simulink model "test_modello"  (R2023a)
settings: Solver=FixedStepAuto  StartTime=0.0  StopTime=50  FixedStep=0.01  RelTol=1e-3
settings Model: PacingRate=0.500000  Creator=kiraa  LastModifiedBy=david
settings OptimizationCC: ReuseModelBlockBuffer=off

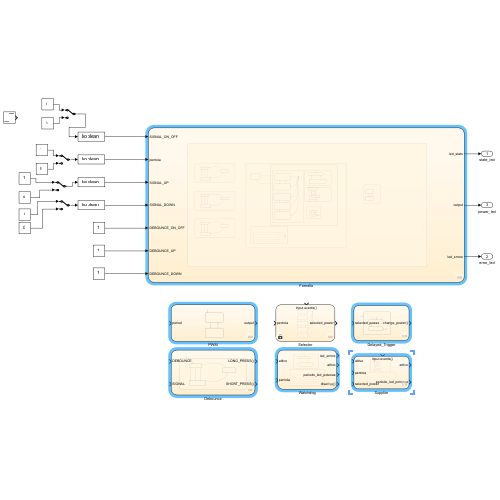
[thumbnail: Simulink's stored preview of the top-level diagram]
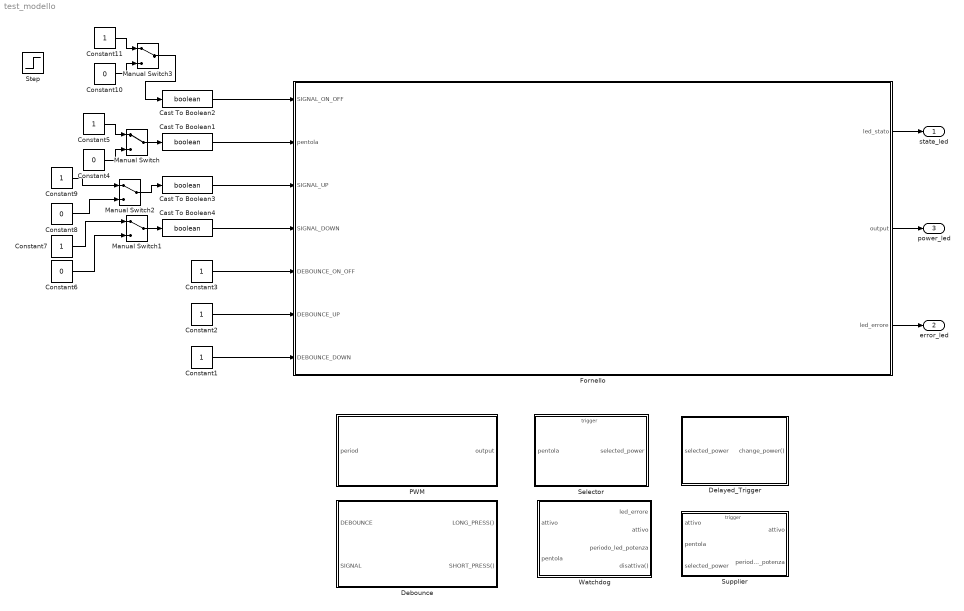
== system test_modello ==
  Cast To Boolean{1..4} (4 alike) : DataTypeConversion  OutDataTypeStr=boolean  RndMeth=Nearest  SaturateOnIntegerOverflow=off
  Constant{1..3,5,7,9,11} (7 alike) : Constant
  Constant{4,6,8,10} (4 alike) : Constant  Value=0
  Debounce : Stateflow chart  TreatAsAtomicUnit=on
  Delayed_Trigger : Stateflow chart  TreatAsAtomicUnit=on
  Fornello : Stateflow chart  TreatAsAtomicUnit=on
  Manual Switch{,1..3} (4 alike) : ManualSwitch
  PWM : Stateflow chart  TreatAsAtomicUnit=on
  Selector : Stateflow chart  TreatAsAtomicUnit=on
  Step : Step  Time=0  SampleTime=0
  Supplier : Stateflow chart  TreatAsAtomicUnit=on
  Watchdog : Stateflow chart  TreatAsAtomicUnit=on
  state_led : Outport
  error_led : Outport  Port=2
  power_led : Outport  Port=3
  wires:
  Manual Switch/1 -> Cast To Boolean1/1
  Fornello/1(led_stato) -> state_led/1
  Fornello/3(led_errore) -> error_led/1
  Constant4/1 -> Manual Switch/2
  Cast To Boolean1/1 -> Fornello/2(pentola)
  Constant1/1 -> Fornello/7(DEBOUNCE_DOWN)
  Constant2/1 -> Fornello/6(DEBOUNCE_UP)
  Constant3/1 -> Fornello/5(DEBOUNCE_ON_OFF)
  Constant5/1 -> Manual Switch/1
  Constant7/1 -> Manual Switch1/1
  Constant6/1 -> Manual Switch1/2
  Constant8/1 -> Manual Switch2/2
  Constant9/1 -> Manual Switch2/1
  Constant11/1 -> Manual Switch3/1
  Constant10/1 -> Manual Switch3/2
  Manual Switch3/1 -> Cast To Boolean2/1
  Cast To Boolean2/1 -> Fornello/1(SIGNAL_ON_OFF)
  Cast To Boolean3/1 -> Fornello/3(SIGNAL_UP)
  Cast To Boolean4/1 -> Fornello/4(SIGNAL_DOWN)
  Manual Switch2/1 -> Cast To Boolean3/1
  Manual Switch1/1 -> Cast To Boolean4/1
  Fornello/2(output) -> power_led/1

== stateflow chart test_modello/Delayed_Trigger ==
  state DELAYED_TRIGGER
    state IDLE
    state DELAYING
    (default) -> IDLE
    IDLE -> DELAYING : [hasChanged(selected_power)]
    DELAYING -> IDLE [order 2] : after(5,sec)/{send(change_power)}
    DELAYING -> DELAYING [order 1] : [hasChanged(selected_power)]
  (default) -> DELAYED_TRIGGER
  data: selected_power input double
  events: change_power output FUNCTION_CALL_EVENT

== stateflow chart test_modello/Fornello ==
  settings: executeAtInitialization=1
  state DEVICE
    state FORNELLO [parallel]
      settings: executionOrder=1
      state ON
        en: led_stato = true
        state SELECTOR [parallel]
          settings: executionOrder=1
          state SELECTED_0W
            en: selected_power=0;
          state SELECTED_300W
            en: selected_power=300;
          state SELECTED_500W
            en: selected_power=500
          state SELECTED_1000W
            en: selected_power=1000
          state SELECTED_1500W
            en: selected_power=1500
          (default) -> SELECTED_0W
          (junction 32) -> SELECTED_0W
          SELECTED_500W -> (junction 32) [order 1] : disattiva
          SELECTED_1000W -> (junction 32) [order 2] : disattiva
          SELECTED_1500W -> (junction 32) [order 2] : disattiva
          SELECTED_300W -> (junction 32) [order 1] : disattiva
          SELECTED_0W -> SELECTED_300W : LONG_PRESS_UP[pentola == false]
          SELECTED_300W -> SELECTED_0W [order 3] : LONG_PRESS_DOWN[pentola==false]
          SELECTED_500W -> SELECTED_300W [order 2] : LONG_PRESS_DOWN[pentola==false]
          SELECTED_300W -> SELECTED_500W [order 2] : LONG_PRESS_UP[pentola == false]
          SELECTED_1000W -> SELECTED_500W [order 3] : LONG_PRESS_DOWN[pentola==false]
          SELECTED_500W -> SELECTED_1000W [order 3] : LONG_PRESS_UP[pentola == false]
          SELECTED_1500W -> SELECTED_1000W [order 1] : LONG_PRESS_DOWN[pentola == false]
          SELECTED_1000W -> SELECTED_1500W [order 1] : LONG_PRESS_UP[pentola==false]
        state WATCHDOG [parallel]
          settings: executionOrder=2
          state IDLE
          state ERROR
            en: led_errore = true
            on after(10,sec): send(disattiva,SELECTOR); erogaPotenza(0)
            ex: led_errore = false
          (default) -> DEVICE.FORNELLO.ON.WATCHDOG.IDLE
          DEVICE.FORNELLO.ON.WATCHDOG.IDLE -> ERROR : [pentola == true && attivo==true]
          ERROR -> DEVICE.FORNELLO.ON.WATCHDOG.IDLE : [pentola == false || attivo == false]
        state SUPPLIER [parallel]
          settings: executionOrder=3
          state NO_CHANGE_REQUESTED
          state Applying_0_power
            en: erogaPotenza(selected_power)
          state Applying_power
            en: erogaPotenza(selected_power)
          state PENDING_CHANGE
          NO_CHANGE_REQUESTED -> PENDING_CHANGE : change_power
          Applying_power -> NO_CHANGE_REQUESTED [order 2]
          Applying_0_power -> NO_CHANGE_REQUESTED
          Applying_power -> Applying_0_power [order 1] : [attivo == false]
          PENDING_CHANGE -> Applying_power : [pentola == false]
        state DELAYED_TRIGGER [parallel]
          settings: executionOrder=4
          state IDLE
          state DELAYING
          (default) -> DEVICE.FORNELLO.ON.DELAYED_TRIGGER.IDLE
          DEVICE.FORNELLO.ON.DELAYED_TRIGGER.IDLE -> DELAYING : change(selected_power)
          DELAYING -> DEVICE.FORNELLO.ON.DELAYED_TRIGGER.IDLE [order 2] : after(5,sec)/{send(change_power, SUPPLIER)}
          DELAYING -> DELAYING [order 1] : change(selected_power)
        (default) -> NO_CHANGE_REQUESTED
      state OFF
        en: led_stato = false; erogaPotenza(0)
      state erogaPotenza(power) [function]
        (default) -> (junction 65) : {power = double(power)}
        (junction 65) -> (junction 68) [order 1] : [power == 0]
        (junction 68) -> (junction 118) : {periodo_led_potenza=0;attivo=false}
        (junction 118) -> (junction 89)
        (junction 65) -> (junction 77) [order 2]
        (junction 77) -> (junction 83) [order 1] : [power == 300]
        (junction 83) -> (junction 120) : {periodo_led_potenza=2;attivo=true}
        (junction 120) -> (junction 89)
        (junction 77) -> (junction 79) [order 2]
        (junction 122) -> (junction 89)
        (junction 119) -> (junction 89)
        (junction 121) -> (junction 89)
        (junction 79) -> (junction 84) [order 1] : [power == 500]
        (junction 84) -> (junction 122) : {periodo_led_potenza=1;attivo=true}
        (junction 79) -> (junction 81) [order 2]
        (junction 81) -> (junction 92) [order 1] : [power == 1000]
        (junction 92) -> (junction 119) : {periodo_led_potenza=0.5;attivo=true}
        (junction 81) -> (junction 95) [order 2]
        (junction 95) -> (junction 99) : [power == 1500]
        (junction 99) -> (junction 121) : {periodo_led_potenza=0.25;attivo=true}
      (default) -> OFF
      OFF -> ON : SHORT_PRESS_ON_OFF
      ON -> OFF : LONG_PRESS_ON_OFF
    state BUTTON_ON_OFF [parallel]
      settings: executionOrder=2
      state HIGH
      state LOW_2
      state LOW
      (default) -> DEVICE.BUTTON_ON_OFF.HIGH
      DEVICE.BUTTON_ON_OFF.LOW_2 -> DEVICE.BUTTON_ON_OFF.HIGH : [SIGNAL_ON_OFF == true]
      DEVICE.BUTTON_ON_OFF.HIGH -> DEVICE.BUTTON_ON_OFF.LOW : [SIGNAL_ON_OFF == false]
      DEVICE.BUTTON_ON_OFF.LOW -> DEVICE.BUTTON_ON_OFF.HIGH [order 2] : before(DEBOUNCE_ON_OFF,sec)[SIGNAL_ON_OFF == true]/{send(SHORT_PRESS_ON_OFF)}
      DEVICE.BUTTON_ON_OFF.LOW -> DEVICE.BUTTON_ON_OFF.HIGH [order 3] : after(DEBOUNCE_ON_OFF,sec)[SIGNAL_ON_OFF == true]/{send(LONG_PRESS_ON_OFF)}
      DEVICE.BUTTON_ON_OFF.LOW -> DEVICE.BUTTON_ON_OFF.LOW_2 [order 1] : after(DEBOUNCE_ON_OFF,sec)[SIGNAL_ON_OFF == false]/{send(LONG_PRESS_ON_OFF)}
    state PWM [parallel]
      settings: executionOrder=5
      state Off
        en: output = false
      state On
        en: output = true
      (default) -> Off
      Off -> On : after(periodo_led_potenza,sec)[periodo_led_potenza ~= 0]
      On -> Off : after(periodo_led_potenza,sec)
    state BUTTON_UP [parallel]
      settings: executionOrder=3
      state HIGH
      state LOW_2
      state LOW
      (default) -> DEVICE.BUTTON_UP.HIGH
      DEVICE.BUTTON_UP.LOW_2 -> DEVICE.BUTTON_UP.HIGH : [SIGNAL_UP == true]
      DEVICE.BUTTON_UP.HIGH -> DEVICE.BUTTON_UP.LOW : [SIGNAL_UP == false]
      DEVICE.BUTTON_UP.LOW -> DEVICE.BUTTON_UP.HIGH [order 2] : before(DEBOUNCE_UP,sec)[SIGNAL_UP == true]/{send(SHORT_PRESS_UP)}
      DEVICE.BUTTON_UP.LOW -> DEVICE.BUTTON_UP.HIGH [order 3] : after(DEBOUNCE_UP,sec)[SIGNAL_UP == true]/{send(LONG_PRESS_UP)}
      DEVICE.BUTTON_UP.LOW -> DEVICE.BUTTON_UP.LOW_2 [order 1] : after(DEBOUNCE_UP,sec)[SIGNAL_UP == false]/{send(LONG_PRESS_UP)}
    state BUTTON_DOWN [parallel]
      settings: executionOrder=4
      state HIGH
      state LOW_2
      state LOW
      (default) -> DEVICE.BUTTON_DOWN.HIGH
      DEVICE.BUTTON_DOWN.LOW_2 -> DEVICE.BUTTON_DOWN.HIGH : [SIGNAL_DOWN == true]
      DEVICE.BUTTON_DOWN.HIGH -> DEVICE.BUTTON_DOWN.LOW : [SIGNAL_DOWN == false]
      DEVICE.BUTTON_DOWN.LOW -> DEVICE.BUTTON_DOWN.HIGH [order 2] : before(DEBOUNCE_DOWN,sec)[SIGNAL_DOWN == true]/{send(SHORT_PRESS_DOWN)}
      DEVICE.BUTTON_DOWN.LOW -> DEVICE.BUTTON_DOWN.HIGH [order 3] : after(DEBOUNCE_DOWN,sec)[SIGNAL_DOWN == true]/{send(LONG_PRESS_DOWN)}
      DEVICE.BUTTON_DOWN.LOW -> DEVICE.BUTTON_DOWN.LOW_2 [order 1] : after(DEBOUNCE_DOWN,sec)[SIGNAL_DOWN == false]/{send(LONG_PRESS_DOWN)}
  (default) -> DEVICE
  data: power function_input double size=1; SIGNAL_ON_OFF input; attivo local boolean size=1 =false; led_stato output boolean size=1 =false; output output; led_errore output boolean size=1 =false; pentola input boolean size=1; SIGNAL_UP input; SIGNAL_DOWN input; DEBOUNCE_ON_OFF input double; DEBOUNCE_UP input double; selected_power local double size=1 =0; DEBOUNCE_DOWN input double; periodo_led_potenza local double size=1 =0
  events: disattiva local FUNCTION_CALL_EVENT; change_power local FUNCTION_CALL_EVENT; LONG_PRESS_DOWN local FUNCTION_CALL_EVENT; LONG_PRESS_UP local FUNCTION_CALL_EVENT; SHORT_PRESS_DOWN local FUNCTION_CALL_EVENT; SHORT_PRESS_UP local FUNCTION_CALL_EVENT; LONG_PRESS_ON_OFF local FUNCTION_CALL_EVENT; SHORT_PRESS_ON_OFF local FUNCTION_CALL_EVENT

== stateflow chart test_modello/Watchdog ==
  state WATCHDOG
    state IDLE
    state ERROR
      en: led_errore = true
      on after(10,sec): send(disattiva); erogaPotenza(0)
      ex: led_errore = false
    (default) -> IDLE
    IDLE -> ERROR : [pentola == true && attivo==true]
    ERROR -> IDLE : [pentola == false || attivo == false]
  state erogaPotenza(power) [function]
    (default) -> (junction 14) : {power = double(power)}
    (junction 14) -> (junction 15) [order 1] : [power == 0]
    (junction 15) -> (junction 16) : {periodo_led_potenza=0;attivo=false}
    (junction 16) -> (junction 20)
    (junction 14) -> (junction 17) [order 2]
    (junction 17) -> (junction 18) [order 1] : [power == 300]
    (junction 18) -> (junction 19) : {periodo_led_potenza=2;attivo=true}
    (junction 19) -> (junction 20)
    (junction 17) -> (junction 21) [order 2]
    (junction 23) -> (junction 20)
    (junction 26) -> (junction 20)
    (junction 29) -> (junction 20)
    (junction 21) -> (junction 22) [order 1] : [power == 500]
    (junction 22) -> (junction 23) : {periodo_led_potenza=1;attivo=true}
    (junction 21) -> (junction 24) [order 2]
    (junction 24) -> (junction 25) [order 1] : [power == 1000]
    (junction 25) -> (junction 26) : {periodo_led_potenza=0.5;attivo=true}
    (junction 24) -> (junction 27) [order 2]
    (junction 27) -> (junction 28) : [power == 1500]
    (junction 28) -> (junction 29) : {periodo_led_potenza=0.25;attivo=true}
  (default) -> WATCHDOG
  data: power function_input double size=1; attivo input boolean; led_errore output boolean; pentola input boolean; attivo output boolean; periodo_led_potenza output double
  events: disattiva output FUNCTION_CALL_EVENT

== stateflow chart test_modello/Supplier ==
  settings: executeAtInitialization=1
  state SUPPLIER
    state NO_CHANGE_REQUESTED
    state Applying_0_power
      en: erogaPotenza(selected_power)
    state Applying_power
      en: erogaPotenza(selected_power)
    state PENDING_CHANGE
    (default) -> NO_CHANGE_REQUESTED
    NO_CHANGE_REQUESTED -> PENDING_CHANGE : change_power
    Applying_power -> NO_CHANGE_REQUESTED [order 2]
    Applying_0_power -> NO_CHANGE_REQUESTED
    Applying_power -> Applying_0_power [order 1] : [attivo == false]
    PENDING_CHANGE -> Applying_power : [pentola==false]
  state erogaPotenza(power) [function]
    (default) -> (junction 19) : {power = double(power)}
    (junction 19) -> (junction 20) [order 1] : [power == 0]
    (junction 20) -> (junction 21) : {periodo_led_potenza=0;attivo=false}
    (junction 21) -> (junction 25)
    (junction 19) -> (junction 22) [order 2]
    (junction 22) -> (junction 23) [order 1] : [power == 300]
    (junction 23) -> (junction 24) : {periodo_led_potenza=2;attivo=true}
    (junction 24) -> (junction 25)
    (junction 22) -> (junction 26) [order 2]
    (junction 28) -> (junction 25)
    (junction 31) -> (junction 25)
    (junction 34) -> (junction 25)
    (junction 26) -> (junction 27) [order 1] : [power == 500]
    (junction 27) -> (junction 28) : {periodo_led_potenza=1;attivo=true}
    (junction 26) -> (junction 29) [order 2]
    (junction 29) -> (junction 30) [order 1] : [power == 1000]
    (junction 30) -> (junction 31) : {periodo_led_potenza=0.5;attivo=true}
    (junction 29) -> (junction 32) [order 2]
    (junction 32) -> (junction 33) : [power == 1500]
    (junction 33) -> (junction 34) : {periodo_led_potenza=0.25;attivo=true}
  (default) -> SUPPLIER
  data: power function_input double size=1; attivo input boolean; pentola input boolean; selected_power input double; attivo output boolean; periodo_led_potenza output double
  events: change_power input FUNCTION_CALL_EVENT; trigger_event input FUNCTION_CALL_EVENT

== stateflow chart test_modello/Selector ==
  state SELECTED_0W
    en: selected_power=0;
  state SELECTED_300W
    en: selected_power=300;
  state SELECTED_500W
    en: selected_power=500
  state SELECTED_1000W
    en: selected_power=1000
  state SELECTED_1500W
    en: selected_power=1500
  (default) -> SELECTED_0W
  (junction 3) -> SELECTED_0W
  SELECTED_500W -> (junction 3) [order 1] : disattiva
  SELECTED_1000W -> (junction 3) [order 2] : disattiva
  SELECTED_1500W -> (junction 3) [order 2] : disattiva
  SELECTED_300W -> (junction 3) [order 1] : disattiva
  SELECTED_0W -> SELECTED_300W : LONG_PRESS_UP[pentola == false]
  SELECTED_300W -> SELECTED_0W [order 3] : LONG_PRESS_DOWN[pentola==false]
  SELECTED_500W -> SELECTED_300W [order 2] : LONG_PRESS_DOWN[pentola==false]
  SELECTED_300W -> SELECTED_500W [order 2] : LONG_PRESS_UP[pentola == false]
  SELECTED_1000W -> SELECTED_500W [order 3] : LONG_PRESS_DOWN[pentola==false]
  SELECTED_500W -> SELECTED_1000W [order 3] : LONG_PRESS_UP[pentola == false]
  SELECTED_1500W -> SELECTED_1000W [order 1] : LONG_PRESS_DOWN[pentola == false]
  SELECTED_1000W -> SELECTED_1500W [order 1] : LONG_PRESS_UP[pentola==false]
  data: pentola input boolean; selected_power output double
  events: LONG_PRESS_DOWN input FUNCTION_CALL_EVENT; LONG_PRESS_UP input FUNCTION_CALL_EVENT; disattiva input FUNCTION_CALL_EVENT; trigger_event input FUNCTION_CALL_EVENT

== stateflow chart test_modello/PWM ==
  state Off
    en: output = false
  state On
    en: output = true
  (default) -> Off
  Off -> On : after(period,sec)[period ~= 0]
  On -> Off : after(period,sec)
  data: output output boolean size=1 =false; period input double size=1

== stateflow chart test_modello/Debounce ==
  state BUTTON
    state HIGH
    state LOW_2
    state LOW
    (default) -> HIGH
    LOW_2 -> HIGH : [SIGNAL == true]
    HIGH -> LOW : [SIGNAL == false]
    LOW -> HIGH [order 2] : before(DEBOUNCE,sec)[SIGNAL == true]/{send(SHORT_PRESS)}
    LOW -> HIGH [order 3] : after(DEBOUNCE,sec)[SIGNAL == true]/{send(LONG_PRESS)}
    LOW -> LOW_2 [order 1] : after(DEBOUNCE,sec)[SIGNAL == false]/{send(LONG_PRESS)}
  (default) -> BUTTON
  data: DEBOUNCE input double; SIGNAL input boolean
  events: LONG_PRESS output FUNCTION_CALL_EVENT; SHORT_PRESS output FUNCTION_CALL_EVENT
